simulink model "Detumbling"  (R2021b)
settings: Solver=VariableStepAuto  StartTime=0.0  StopTime=10.0  RelTol=1e-3
settings Model: Creator=jorgemarrero  LastModifiedBy=jorgemarrero

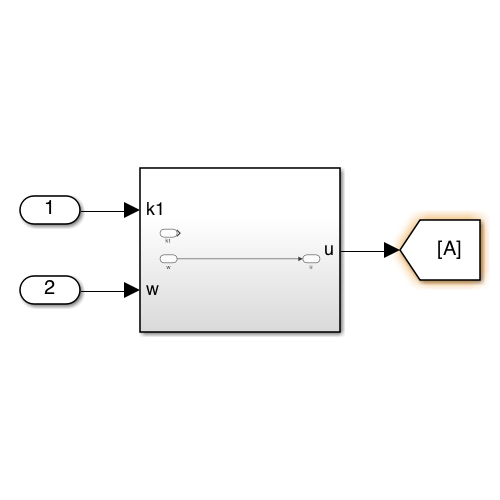
[thumbnail: Simulink's stored preview of the top-level diagram]
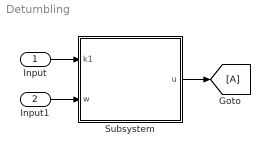
== system Detumbling ==
  Input : Inport
  Input1 : Inport  Port=2
  Subsystem : Subsystem
  wires:
  Input1/1 -> Subsystem/2(w)
  Input/1 -> Subsystem/1(k1)
  Subsystem/1(u) -> [A]

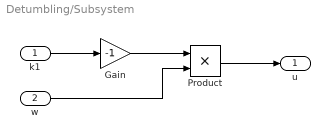
== system Detumbling/Subsystem ==
  k1 : Inport
  w : Inport  Port=2
  Gain : Gain  Gain=-1
  Product : Product
  u : Outport
  wires:
  w/1 -> Product/2
  k1/1 -> Gain/1
  Gain/1 -> Product/1
  Product/1 -> u/1
